simulink model "prvi_filtar_simulink"  (Simulink 7.6)
settings: Solver=ode45  StartTime=0.0  StopTime=15000  MaxStep=1  RelTol=1e-3
libraries: simulink x4
settings Model: Creator=Ogi  LastModifiedBy=Ogi

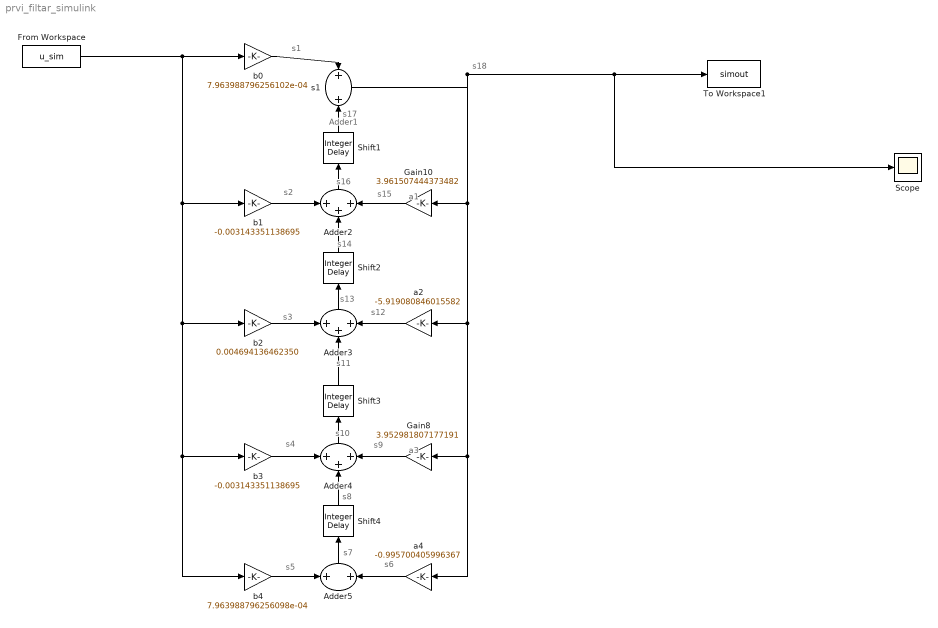
== system prvi_filtar_simulink ==
  note: Adder1
  note: a1
  note: a3
  note: s1
  note: s2
  note: s3
  note: s4
  note: s5
  note: s6
  note: s7
  note: s8
  note: s10
  note: s11
  note: s13
  note: s14
  note: s16
  note: s17
  note: s18
  note: s9
  note: s12
  note: s15
  Adder2 : Sum  Inputs=+++  OutDataTypeStr=fixdt(1, x, y)  RndMeth=Nearest
  Adder3 : Sum  Inputs=+++  OutDataTypeStr=fixdt(1, x, y)  RndMeth=Nearest
  Adder4 : Sum  Inputs=+++  OutDataTypeStr=fixdt(1, x, y)  RndMeth=Nearest
  Adder5 : Sum  OutDataTypeStr=fixdt(1, x, y)  RndMeth=Nearest
  From Workspace : FromWorkspace  VariableName=u_sim
  Gain10 : Gain  Gain=3.961507444373482  ParamDataTypeStr=fixdt(1, j, k)  OutDataTypeStr=fixdt(1, x, y)  RndMeth=Nearest
  Gain8 : Gain  Gain=3.952981807177191  ParamDataTypeStr=fixdt(1, j, k)  OutDataTypeStr=fixdt(1, x, y)  RndMeth=Nearest
  Scope : Scope
  Shift{1..4} (4 alike) : simulink/Discrete/Integer Delay  NumDelays=1  vinit=0.0  samptime=-1
  To Workspace1 : ToWorkspace  VariableName=simout  SampleTime=-1  SaveFormat=Array
  a2 : Gain  Gain=-5.919080846015582  ParamDataTypeStr=fixdt(1, j, k)  OutDataTypeStr=fixdt(1, x, y)  RndMeth=Nearest
  a4 : Gain  Gain=-0.995700405996367  ParamDataTypeStr=fixdt(1, j, k)  OutDataTypeStr=fixdt(1, x, y)  RndMeth=Nearest
  b0 : Gain  Gain=7.963988796256102e-04  ParamDataTypeStr=fixdt(1, j, k)  OutDataTypeStr=fixdt(1, x, y)  RndMeth=Nearest
  b1 : Gain  Gain=-0.003143351138695  ParamDataTypeStr=fixdt(1, j, k)  OutDataTypeStr=fixdt(1, x, y)  RndMeth=Nearest
  b2 : Gain  Gain=0.004694136462350  ParamDataTypeStr=fixdt(1, j, k)  OutDataTypeStr=fixdt(1, x, y)  RndMeth=Nearest
  b3 : Gain  Gain=-0.003143351138695  ParamDataTypeStr=fixdt(1, j, k)  OutDataTypeStr=fixdt(1, x, y)  RndMeth=Nearest
  b4 : Gain  Gain=7.963988796256098e-04  ParamDataTypeStr=fixdt(1, j, k)  OutDataTypeStr=fixdt(1, x, y)  RndMeth=Nearest
  s1 : Sum  OutDataTypeStr=fixdt(1, x, y)  RndMeth=Nearest
  wires:
  Adder3/1 -> Shift2/1
  b1/1 -> Adder2/1
  Shift2/1 -> Adder2/2
  Gain10/1 -> Adder2/3
  Adder2/1 -> Shift1/1
  Shift1/1 -> s1/2
  s1/1 -> Gain10/1, a2/1, Gain8/1, a4/1, Scope/1, To Workspace1/1
  Adder5/1 -> Shift4/1
  b3/1 -> Adder4/1
  Shift4/1 -> Adder4/2
  Gain8/1 -> Adder4/3
  Adder4/1 -> Shift3/1
  a4/1 -> Adder5/2
  Shift3/1 -> Adder3/2
  a2/1 -> Adder3/3
  b2/1 -> Adder3/1
  b4/1 -> Adder5/1
  b0/1 -> s1/1
  From Workspace/1 -> b2/1, b4/1, b3/1, b1/1, b0/1
